simulink model "test_2"  (R2025b)
settings: Solver=FixedStepDiscrete  StartTime=0.0  StopTime=inf  RelTol=1e-3
libraries: instrumentlib x1
settings Model: Creator=Albert  LastModifiedBy=Albert

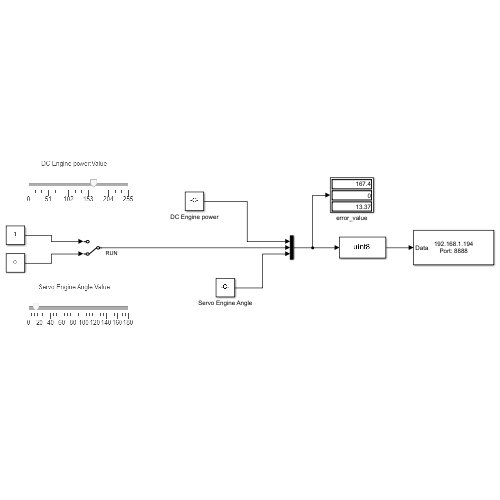
[thumbnail: Simulink's stored preview of the top-level diagram]
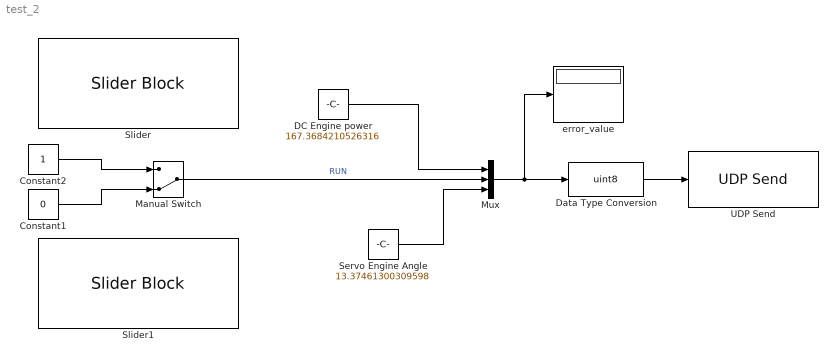
== system test_2 ==
  Constant1 : Constant  Value=0
  Constant2 : Constant
  DC Engine power : Constant  Value=167.3684210526316
  Data Type Conversion : DataTypeConversion  OutDataTypeStr=uint8  SaturateOnIntegerOverflow=off  RndMeth=Floor
  Manual Switch : ManualSwitch  CurrentSetting=0
  Mux : Mux  Inputs=3
  Servo Engine Angle : Constant  Value=13.37461300309598
  Slider : SliderBlock  ScaleMax=255
  Slider1 : SliderBlock  ScaleMax=180
  UDP Send : instrumentlib/UDP Send  Host=192.168.1.194  Port=8888  LocalAddress=0.0.0.0  LocalPort=-1  EnablePortSharing=off  OutputDatagramPacketSize=512  ByteOrder=little-endian  EnableBlockingMode=on  SimulateUsing=Interpreted execution
  error_value : Display
  wires:
  Data Type Conversion/1 -> UDP Send/1
  Constant2/1 -> Manual Switch/1
  Constant1/1 -> Manual Switch/2
  Mux/1 -> error_value/1, Data Type Conversion/1
  DC Engine power/1 -> Mux/1
  Servo Engine Angle/1 -> Mux/3
  Manual Switch/1 -> Mux/2  "RUN"
